simulink model "LMS_adaptation"  (R2014b)
settings: Solver=ode45  StartTime=0.0  StopTime=500e-9  RelTol=1e-3
libraries: ams_primitives x4
settings Model: Creator=Jase  LastModifiedBy=Jase
settings DataIOCC: InspectSignalLogs=on

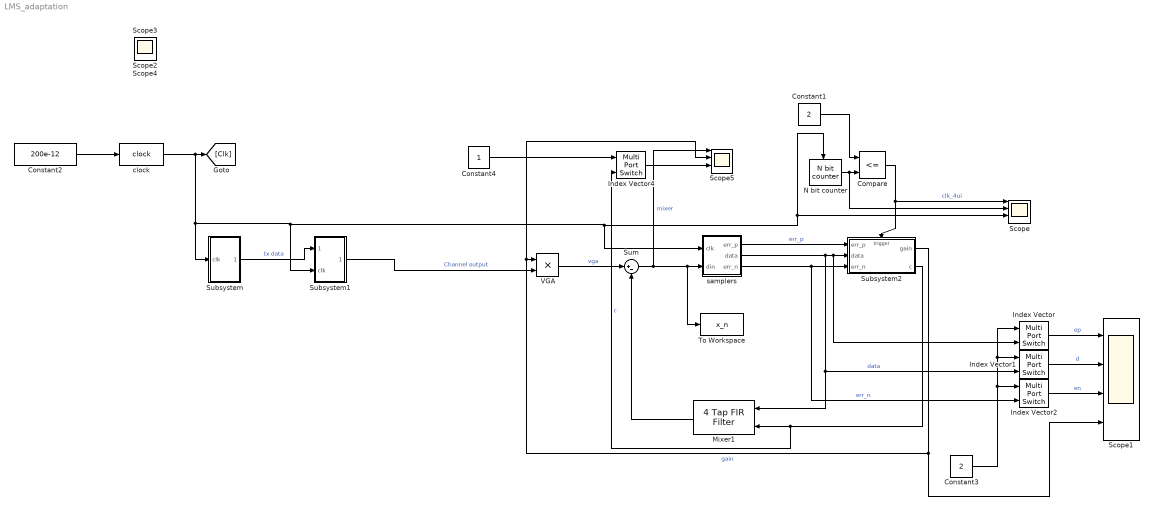
== system LMS_adaptation ==
  Compare : RelationalOperator  Operator=<=  OutDataTypeStr=boolean  InputSameDT=on
  Constant1 : Constant  Value=2
  Constant2 : Constant  Value=200e-12
  Constant3 : Constant  Value=2
  Constant4 : Constant
  Index Vector{,1..2,4} (4 alike) : MultiPortSwitch  DataPortOrder=Zero-based contiguous  Inputs=1  zeroidx=on
  Mixer1 : ams_primitives/4 Tap FIR Filter
  N bit counter : ams_primitives/N bit counter  N=4
  Scope{,1,3,5} (4 alike) : Scope  NumInputPorts=4
      Scope settings: YMin=-5~-5~-5~-5  YMax=5~5~5~5
      Scope1 settings: ShowLegends=on  YMin=-5~-5~-5~-5  YMax=5~5~5~5
      Scope5 settings: YMin=-0.1~0~-1~-1  YMax=0.05~0.06~1~1  SaveName=ScopeData6
      Scope3 settings: SaveName=ScopeData4
  Subsystem : Subsystem
  Subsystem1 : Subsystem
  Subsystem2 : Subsystem
  Sum : Sum  Inputs=|+-
  To Workspace : ToWorkspace  VariableName=x_n  SampleTime=-1
  VGA : Product
  "clock " : ams_primitives/clock 
  samplers : Subsystem
  Scope2 : Scope
      settings: SaveName=ScopeData2
  Scope4 : Scope
      settings: SaveName=ScopeData5
  wires:
  Subsystem/1(Out1) -> Subsystem1/1(In1)  "tx data"
  Subsystem1/1(x(t)) -> VGA/2  "Channel output"
  Constant2/1 -> "clock "/1
  "clock "/1 -> Scope/3, N bit counter/Trigger, samplers/1(clk), Subsystem1/2(clk), Subsystem/1(clk), [Clk]
  VGA/1 -> Sum/1  "vga"
  Mixer1/1 -> Sum/2
  samplers/2(data) -> Index Vector1/2, Mixer1/1, Index Vector/2, Subsystem2/2(data)  "data"
  Sum/1 -> Scope5/1, To Workspace/1, samplers/2(din)  "mixer"
  samplers/1(err_p) -> Subsystem2/1(err_p)  "err_p"
  samplers/3(err_n) -> Index Vector2/2, Subsystem2/3(err_n)  "err_n"
  Subsystem2/1(gain) -> Scope1/4, Scope5/2, VGA/1  "gain"
  Subsystem2/2(c) -> Index Vector4/2, Mixer1/2  "c"
  N bit counter/1 -> Scope/2, Compare/2
  Compare/1 -> Subsystem2/Trigger, Scope/1  "clk_4ui"
  Constant1/1 -> Compare/1
  Index Vector/1 -> Scope1/1  "ep"
  Index Vector1/1 -> Scope1/2  "d"
  Index Vector2/1 -> Scope1/3  "en"
  Constant3/1 -> Index Vector2/1, Index Vector1/1, Index Vector/1
  Index Vector4/1 -> Scope5/3
  Constant4/1 -> Index Vector4/1

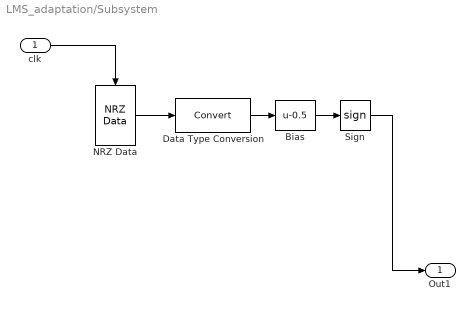
== system LMS_adaptation/Subsystem ==
  clk : Inport
  Bias : Bias  Bias=-0.5
  Data Type Conversion : DataTypeConversion
  NRZ Data : ams_primitives/NRZ Data
  Sign : Signum
  Out1 : Outport
  wires:
  Data Type Conversion/1 -> Bias/1
  NRZ Data/1 -> Data Type Conversion/1
  Sign/1 -> Out1/1
  Bias/1 -> Sign/1
  clk/1 -> NRZ Data/Trigger

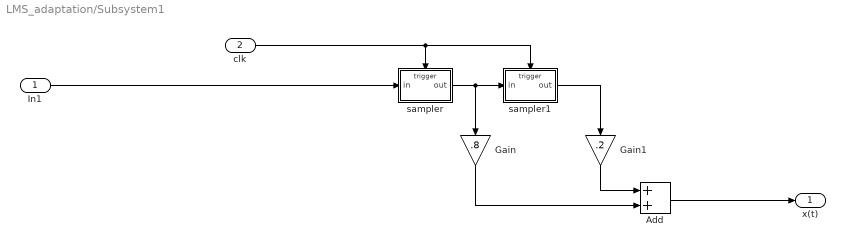
== system LMS_adaptation/Subsystem1 ==
  In1 : Inport
  clk : Inport  Port=2
  Add : Sum
  Gain : Gain  Gain=.8
  Gain1 : Gain  Gain=.2
  sampler : Subsystem
  sampler1 : Subsystem
  x(t) : Outport
  wires:
  clk/1 -> sampler1/Trigger, sampler/Trigger
  Add/1 -> x(t)/1
  Gain1/1 -> Add/1
  Gain/1 -> Add/2
  sampler/1(out) -> sampler1/1(in), Gain/1
  sampler1/1(out) -> Gain1/1
  In1/1 -> sampler/1(in)

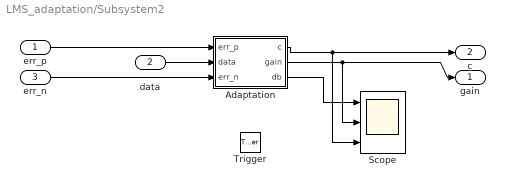
== system LMS_adaptation/Subsystem2 ==
  err_p : Inport  LatchByDelayingOutsideSignal=on
  data : Inport  Port=2  LatchByDelayingOutsideSignal=on
  err_n : Inport  Port=3  LatchByDelayingOutsideSignal=on
  Trigger : TriggerPort  PortDimensions=1
  Adaptation : MATLAB Function  TreatAsAtomicUnit=on
  Scope : Scope  NumInputPorts=3
      settings: YMin=0~-1.5~-0.5  YMax=1~1~0.1  SaveName=ScopeData3
  gain : Outport
  c : Outport  Port=2
  wires:
  Adaptation/2(gain) -> Scope/2, gain/1
  Adaptation/1(c) -> Scope/3, c/1
  err_n/1 -> Adaptation/3(err_n)
  err_p/1 -> Adaptation/1(err_p)
  data/1 -> Adaptation/2(data)
  Adaptation/3(db) -> Scope/1

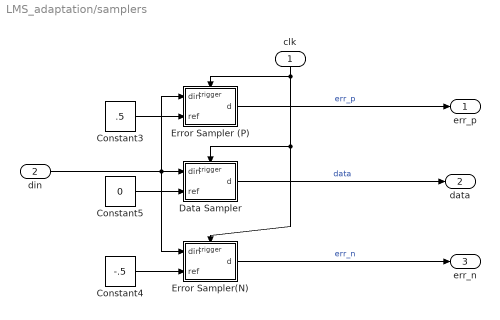
== system LMS_adaptation/samplers ==
  clk : Inport
  din : Inport  Port=2
  Constant3 : Constant  Value=.5
  Constant4 : Constant  Value=-.5
  Constant5 : Constant  Value=0
  Data Sampler : Subsystem
  Error Sampler (P) : Subsystem
  Error Sampler(N) : Subsystem
  err_p : Outport
  data : Outport  Port=2
  err_n : Outport  Port=3
  wires:
  din/1 -> Error Sampler(N)/1(din), Error Sampler (P)/1(din), Data Sampler/1(din)
  Data Sampler/1(d) -> data/1  "data"
  Constant4/1 -> Error Sampler(N)/2(ref)
  Error Sampler(N)/1(d) -> err_n/1  "err_n"
  Error Sampler (P)/1(d) -> err_p/1  "err_p"
  Constant3/1 -> Error Sampler (P)/2(ref)
  Constant5/1 -> Data Sampler/2(ref)
  clk/1 -> Data Sampler/Trigger, Error Sampler(N)/Trigger, Error Sampler (P)/Trigger

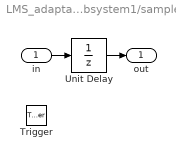
== system LMS_adaptation/Subsystem1/sampler ==
  in : Inport
  Trigger : TriggerPort  PortDimensions=1
  Unit Delay : UnitDelay  SampleTime=-1
  out : Outport
  wires:
  in/1 -> Unit Delay/1
  Unit Delay/1 -> out/1

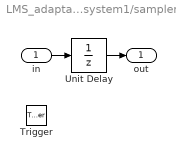
== system LMS_adaptation/Subsystem1/sampler1 ==
  in : Inport
  Trigger : TriggerPort  PortDimensions=1
  Unit Delay : UnitDelay  SampleTime=-1
  out : Outport
  wires:
  Unit Delay/1 -> out/1
  in/1 -> Unit Delay/1

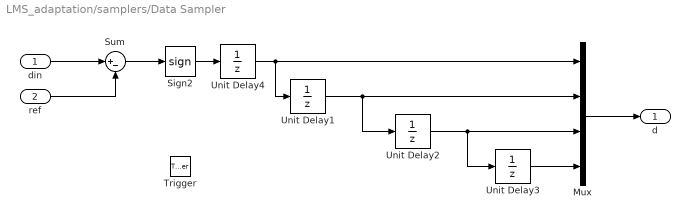
== system LMS_adaptation/samplers/Data Sampler ==
  din : Inport  LatchByDelayingOutsideSignal=on
  ref : Inport  Port=2
  Trigger : TriggerPort  PortDimensions=1
  Mux : Mux
  Sign2 : Signum
  Sum : Sum  Inputs=|+-
  Unit Delay{1..4} (4 alike) : UnitDelay  SampleTime=-1
  d : Outport
  wires:
  Unit Delay1/1 -> Mux/2, Unit Delay2/1
  Unit Delay2/1 -> Mux/3, Unit Delay3/1
  Unit Delay3/1 -> Mux/4
  Mux/1 -> d/1
  Sign2/1 -> Unit Delay4/1
  Unit Delay4/1 -> Mux/1, Unit Delay1/1
  din/1 -> Sum/1
  Sum/1 -> Sign2/1
  ref/1 -> Sum/2

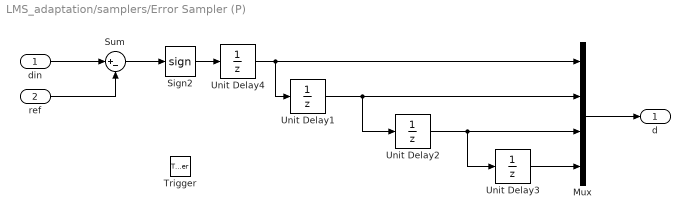
== system LMS_adaptation/samplers/Error Sampler (P) ==
  din : Inport
  ref : Inport  Port=2
  Trigger : TriggerPort  PortDimensions=1
  Mux : Mux
  Sign2 : Signum
  Sum : Sum  Inputs=|+-
  Unit Delay{1..4} (4 alike) : UnitDelay  SampleTime=-1
  d : Outport
  wires:
  ref/1 -> Sum/2
  Sum/1 -> Sign2/1
  din/1 -> Sum/1
  Unit Delay4/1 -> Unit Delay1/1, Mux/1
  Sign2/1 -> Unit Delay4/1
  Mux/1 -> d/1
  Unit Delay3/1 -> Mux/4
  Unit Delay2/1 -> Unit Delay3/1, Mux/3
  Unit Delay1/1 -> Unit Delay2/1, Mux/2

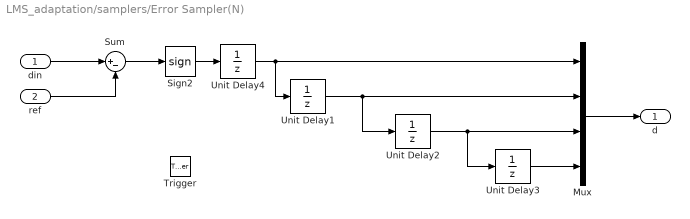
== system LMS_adaptation/samplers/Error Sampler(N) ==
  din : Inport
  ref : Inport  Port=2
  Trigger : TriggerPort  PortDimensions=1
  Mux : Mux
  Sign2 : Signum
  Sum : Sum  Inputs=|+-
  Unit Delay{1..4} (4 alike) : UnitDelay  SampleTime=-1
  d : Outport
  wires:
  Unit Delay1/1 -> Mux/2, Unit Delay2/1
  Unit Delay2/1 -> Mux/3, Unit Delay3/1
  Unit Delay3/1 -> Mux/4
  Mux/1 -> d/1
  Sign2/1 -> Unit Delay4/1
  Unit Delay4/1 -> Mux/1, Unit Delay1/1
  din/1 -> Sum/1
  Sum/1 -> Sign2/1
  ref/1 -> Sum/2

== matlab function LMS_adaptation/Subsystem2/Adaptation ==
  data: err_p input; c output; data input; err_n input; gain output; db output
function [c, gain, db] = fcn(err_p, data, err_n)
%#codegen
persistent c_ gain_ mu;

if isempty(c_)
    c_ = [0. 0. 0. 0.]';
    gain_ = 0.5;
    mu = .01;
end

% Compute gain coefficient
% e_p    d   e_n | gain   c
% ------------------------
%   0    0   0   | -1     
%   0    1   1   | +1
%   1    1   1   | -1
%   0    0   1   | +1

d_cmos = 0.5*(data+1);
gain_adj = -1*d_cmos.*err_p + ~d_cmos.*err_n;

c_ = c_ + mu*(-1*d_cmos.*err_p + ~d_cmos.*err_n);

err = (d_cmos(1)*err_p + ~d_cmos(1)*err_n);

c_ = c_ + mu*(-1*d_cmos.*err + ~d_cmos.*err);

% Majority vote
g = sum(gain_adj) > 1;

% Gain calculation
gain_ = gain_ + g*mu + -1*~g*mu;

db = sum(gain_adj);
c = [c_(1) 0 0 0];
gain = gain_*.1;
